simulink model "DriveTrainFinal"  (R2020b)
settings: Solver=VariableStepAuto  StartTime=0.0  StopTime=155  MaxStep=0.001  MinStep=0.0001  RelTol=1e-3
undefined symbols (not defined in the file): magnitude
libraries: simulink x3
settings Model: EnablePacing=on  Creator=markb  LastModifiedBy=orangejuzi
settings SolverCC: AlgebraicLoopSolver=LineSearch

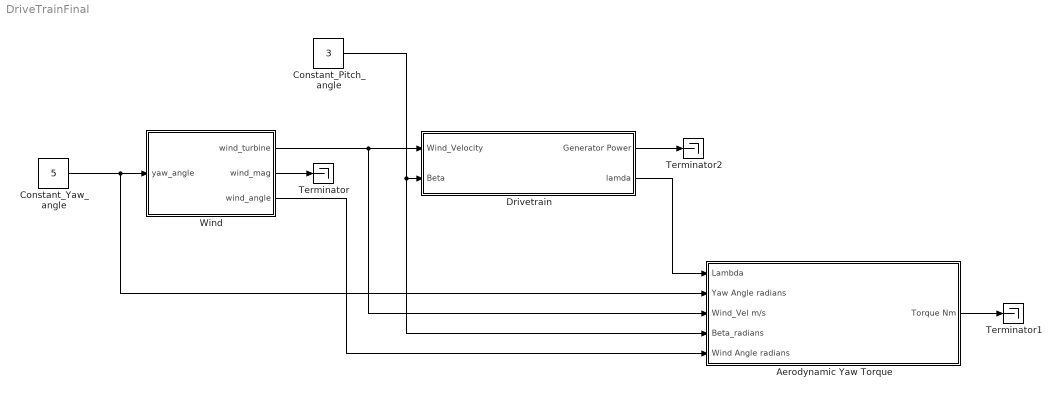
== system DriveTrainFinal ==
  Aerodynamic Yaw Torque : Subsystem
  Constant_Pitch_angle : Constant  Value=3
  Constant_Yaw_angle : Constant  Value=5
  Drivetrain : Subsystem
  Terminator : Terminator
  Terminator1 : Terminator
  Terminator2 : Terminator
  Wind : Subsystem
  wires:
  Wind/1(wind_turbine) -> Aerodynamic Yaw Torque/3(Wind_Vel m/s), Drivetrain/1(Wind_Velocity)
  Constant_Yaw_angle/1 -> Aerodynamic Yaw Torque/2(Yaw Angle radians), Wind/1(yaw_angle)
  Wind/2(wind_mag) -> Terminator/1
  Wind/3(wind_angle) -> Aerodynamic Yaw Torque/5(Wind Angle radians)
  Constant_Pitch_angle/1 -> Aerodynamic Yaw Torque/4(Beta_radians), Drivetrain/2(Beta)
  Drivetrain/1(Generator Power) -> Terminator2/1
  Drivetrain/2(lamda) -> Aerodynamic Yaw Torque/1(Lambda)
  Aerodynamic Yaw Torque/1(Torque Nm) -> Terminator1/1

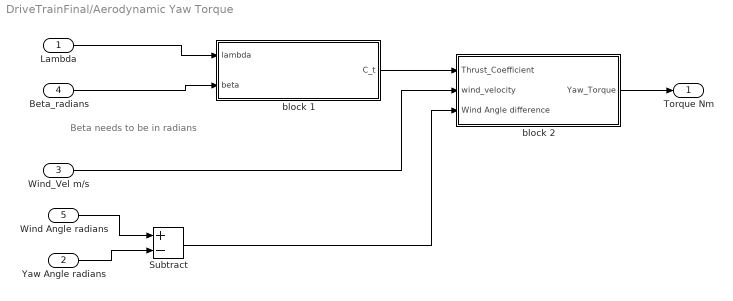
== system DriveTrainFinal/Aerodynamic Yaw Torque ==
  note: Beta needs to be in radians
  Lambda : Inport
  Yaw Angle radians : Inport  Port=2
  Wind_Vel m/s : Inport  Port=3
  Beta_radians : Inport  Port=4
  Wind Angle radians : Inport  Port=5
  Subtract : Sum  Inputs=+-
  block 1 : Subsystem
  block 2 : Subsystem
  Torque Nm : Outport
  wires:
  block 1/1(C_t) -> block 2/1(Thrust_Coefficient)
  Beta_radians/1 -> block 1/2(beta)
  Wind Angle radians/1 -> Subtract/1
  Yaw Angle radians/1 -> Subtract/2
  Subtract/1 -> block 2/3(Wind Angle difference)
  block 2/1(Yaw_Torque) -> Torque Nm/1
  Lambda/1 -> block 1/1(lambda)
  Wind_Vel m/s/1 -> block 2/2(wind_velocity)

== system DriveTrainFinal/Drivetrain ==
  Wind_Velocity : Inport
  Beta : Inport  Port=2
  Aerodynamic Block : Subsystem
  Electricl Block : Subsystem
  Mechanical Bock : Subsystem
  Generator Power : Outport
  lamda : Outport  Port=2
  wires:
  Mechanical Bock/2(omega_Gen) -> Electricl Block/1(HSS_Speed)
  Electricl Block/2(Generator Torque) -> Mechanical Bock/2(Gen_Torque)
  Mechanical Bock/1(omega_rotor) -> Aerodynamic Block/1(Rotor_Angular_Velocity)
  Wind_Velocity/1 -> Aerodynamic Block/2(Wind_Velocity)
  Beta/1 -> Aerodynamic Block/3(Beta)
  Aerodynamic Block/2(lamda) -> lamda/1
  Aerodynamic Block/1(Rotor_Torque) -> Mechanical Bock/1(Rotor_Torque)
  Electricl Block/1(Generator Power) -> Generator Power/1

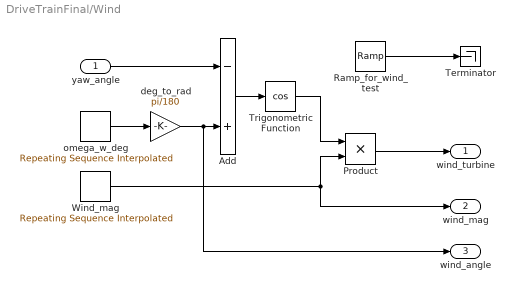
== system DriveTrainFinal/Wind ==
  yaw_angle : Inport
  Add : Sum  Inputs=-+
  Product : Product
  Ramp_for_wind_test : simulink/Sources/Ramp  slope=0.1  start=0  InitialOutput=10
  Terminator : Terminator
  Trigonometric Function : Trigonometry  Operator=cos
  Wind_mag : simulink/Sources/Repeating Sequence Interpolated  OutValues=[6 10 15 10 10 15 18 20 22 26 20 22 18 15 13 13 12 10 9 11 17 17 19 19 25 25 26 19 13 10 7 ].'  TimeValues=[0 5 15 20 25 30 35 40 45 50 55 60 65 70 75 80 85 90 95 100 105 110 115 120 125 130 135 140 145 150 155 ].'  LookUpMeth=Interpolation-Use End Values  tsamp=0.01  OutMin=[]  OutMax=[]  OutDataTypeStr=double  OutputDataTypeScalingMode=double  OutDataType=fixdt(0,8)  OutScaling=2^-10
  deg_to_rad : Gain  Gain=pi/180
  omega_w_deg : simulink/Sources/Repeating Sequence Interpolated  OutValues=[ 0 0 0 6 10 12 12 4 8 12 16 16 24 28 24 16 12 4 2 0 0 -2 -4 -4 -10 -14 -18 -20 -12 -8 -4 ].'  TimeValues=[0 5 15 20 25 30 35 40 45 50 55 60 65 70 75 80 85 90 95 100 105 110 115 120 125 130 135 140 145 150 155 ].'  LookUpMeth=Interpolation-Use End Values  tsamp=0.01  OutMin=[]  OutMax=[]  OutDataTypeStr=double  OutputDataTypeScalingMode=double  OutDataType=fixdt(0,8)  OutScaling=2^-10
  wind_turbine : Outport
  wind_mag : Outport  Port=2
  wind_angle : Outport  Port=3
  wires:
  Add/1 -> Trigonometric Function/1
  Trigonometric Function/1 -> Product/1
  deg_to_rad/1 -> wind_angle/1, Add/2
  yaw_angle/1 -> Add/1
  omega_w_deg/1 -> deg_to_rad/1
  Wind_mag/1 -> wind_mag/1, Product/2
  Product/1 -> wind_turbine/1
  Ramp_for_wind_test/1 -> Terminator/1

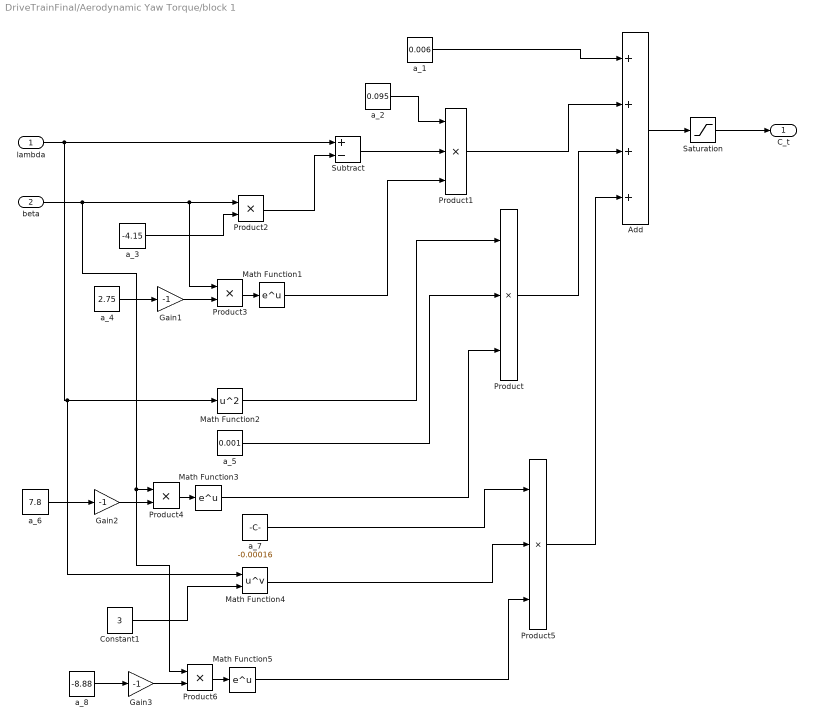
== system DriveTrainFinal/Aerodynamic Yaw Torque/block 1 ==
  lambda : Inport
  beta : Inport  Port=2
  Add : Sum  Inputs=++++
  Constant1 : Constant  Value=3
  Gain1 : Gain  Gain=-1
  Gain2 : Gain  Gain=-1
  Gain3 : Gain  Gain=-1
  Math Function1 : Math  SaturateOnIntegerOverflow=on
  Math Function2 : Math  Operator=square  SaturateOnIntegerOverflow=on
  Math Function3 : Math  SaturateOnIntegerOverflow=on
  Math Function4 : Math  Operator=pow  SaturateOnIntegerOverflow=on
  Math Function5 : Math  SaturateOnIntegerOverflow=on
  Product : Product  Inputs=3
  Product1 : Product  Inputs=3
  Product{2..4,6} (4 alike) : Product
  Product5 : Product  Inputs=3
  Saturation : Saturate  UpperLimit=inf  LowerLimit=0
  Subtract : Sum  Inputs=+-
  a_1 : Constant  Value=0.006
  a_2 : Constant  Value=0.095
  a_3 : Constant  Value=-4.15
  a_4 : Constant  Value=2.75
  a_5 : Constant  Value=0.001
  a_6 : Constant  Value=7.8
  a_7 : Constant  Value=-0.00016
  a_8 : Constant  Value=-8.88
  C_t : Outport
  wires:
  a_3/1 -> Product2/2
  beta/1 -> Product6/1, Product4/1, Product2/1, Product3/1
  a_1/1 -> Add/1
  Product1/1 -> Add/2
  Math Function5/1 -> Product5/3
  Gain3/1 -> Product6/2
  lambda/1 -> Math Function4/1, Math Function2/1, Subtract/1
  Math Function2/1 -> Product/1
  a_4/1 -> Gain1/1
  Product5/1 -> Add/4
  a_2/1 -> Product1/1
  Product3/1 -> Math Function1/1
  Product6/1 -> Math Function5/1
  Product4/1 -> Math Function3/1
  Math Function1/1 -> Product1/3
  Constant1/1 -> Math Function4/2
  Math Function4/1 -> Product5/2
  a_5/1 -> Product/2
  Add/1 -> Saturation/1
  Product2/1 -> Subtract/2
  Subtract/1 -> Product1/2
  Gain1/1 -> Product3/2
  a_7/1 -> Product5/1
  a_8/1 -> Gain3/1
  Gain2/1 -> Product4/2
  Math Function3/1 -> Product/3
  Product/1 -> Add/3
  a_6/1 -> Gain2/1
  Saturation/1 -> C_t/1

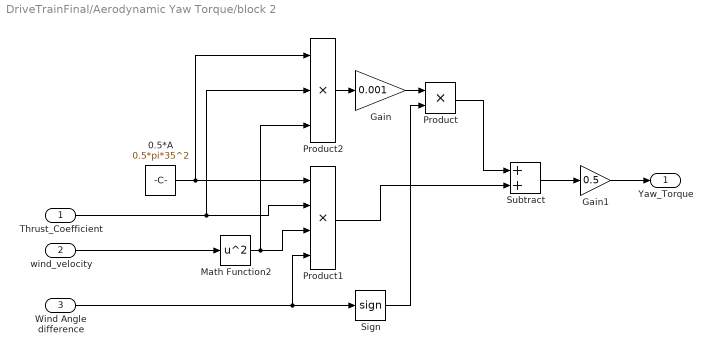
== system DriveTrainFinal/Aerodynamic Yaw Torque/block 2 ==
  Thrust_Coefficient : Inport
  wind_velocity : Inport  Port=2
  Wind Angle difference : Inport  Port=3
  0.5*A : Constant  Value=0.5*pi*35^2
  Gain : Gain  Gain=0.001
  Gain1 : Gain  Gain=0.5
  Math Function2 : Math  Operator=square  SaturateOnIntegerOverflow=on
  Product : Product
  Product1 : Product  Inputs=4
  Product2 : Product  Inputs=3
  Sign : Signum
  Subtract : Sum
  Yaw_Torque : Outport
  wires:
  0.5*A/1 -> Product2/1, Product1/1
  Thrust_Coefficient/1 -> Product2/2, Product1/2
  Math Function2/1 -> Product2/3, Product1/3
  wind_velocity/1 -> Math Function2/1
  Wind Angle difference/1 -> Product1/4, Sign/1
  Product2/1 -> Gain/1
  Product1/1 -> Subtract/2
  Subtract/1 -> Gain1/1
  Gain/1 -> Product/1
  Sign/1 -> Product/2
  Product/1 -> Subtract/1
  Gain1/1 -> Yaw_Torque/1

== system DriveTrainFinal/Drivetrain/Aerodynamic Block ==
  Rotor_Angular_Velocity : Inport
  Wind_Velocity : Inport  Port=2
  Beta : Inport  Port=3
  Power Coefficient : Subsystem
  Rotor Torque : Subsystem
  Tip speed Ratio : Subsystem
  Rotor_Torque : Outport
  lamda : Outport  Port=2
  wires:
  Beta/1 -> Power Coefficient/2(Beta)
  Tip speed Ratio/1(Tip_Speed_Ratio) -> lamda/1, Power Coefficient/1(Lamda)
  Power Coefficient/1(C_p) -> Rotor Torque/1(Power_Coefficient)
  Rotor_Angular_Velocity/1 -> Rotor Torque/3(Rotor_Angular_Velocity), Tip speed Ratio/1(Rotor_Angular_Velocity)
  Rotor Torque/1(Rotor_Torque) -> Rotor_Torque/1
  Wind_Velocity/1 -> Rotor Torque/2(Wind_Speed), Tip speed Ratio/2(Wind_Velocity)

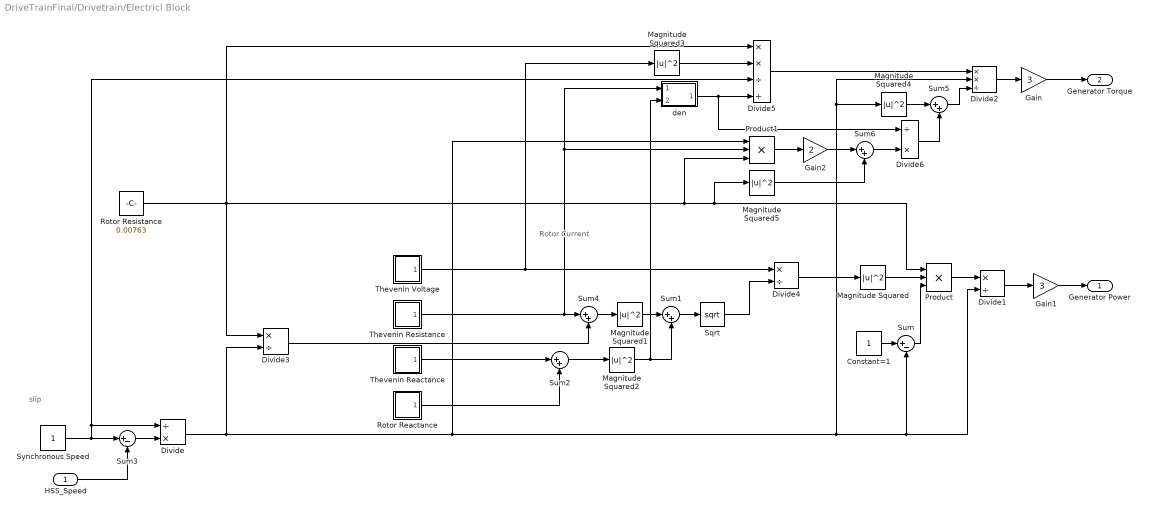
== system DriveTrainFinal/Drivetrain/Electricl Block ==
  note: slip
  note: Rotor Current
  HSS_Speed : Inport
  Constant=1 : Constant
  Divide : Product  Inputs=/*
  Divide1 : Product  Inputs=*/
  Divide2 : Product  Inputs=**/
  Divide3 : Product  Inputs=*/
  Divide4 : Product  Inputs=*/
  Divide5 : Product  Inputs=**//
  Divide6 : Product  Inputs=/*
  Gain : Gain  Gain=3
  Gain1 : Gain  Gain=3
  Gain2 : Gain  Gain=2
  Magnitude Squared{,1..5} (6 alike) : Math  Operator=magnitude^2  SaturateOnIntegerOverflow=on
  Product : Product  Inputs=3
  Product1 : Product  Inputs=3
  Rotor Reactance : Subsystem
  Rotor Resistance : Constant  Value=0.00763
  Sqrt : Sqrt  SaturateOnIntegerOverflow=on
  Sum : Sum  Inputs=|+-
  Sum{1..2,4..6} (5 alike) : Sum  Inputs=|++
  Sum3 : Sum  Inputs=|+-
  Synchronous Speed : Constant
  Thevenin Reactance : Subsystem
  Thevenin Resistance : Subsystem
  Thevenin Voltage : Subsystem
  den : Subsystem
  Generator Power : Outport
  Generator Torque : Outport  Port=2
  wires:
  Product/1 -> Divide1/1
  Divide1/1 -> Gain1/1
  Gain1/1 -> Generator Power/1
  Sum/1 -> Product/3
  Divide/1 -> Product1/1, Divide1/2, Sum/2, Divide2/2, Magnitude Squared4/1, Divide3/2
  Constant=1/1 -> Sum/1
  Rotor Resistance/1 -> Product1/3, Product/1, Magnitude Squared5/1, Divide3/1, Divide5/1
  Divide4/1 -> Magnitude Squared/1
  Magnitude Squared/1 -> Product/2
  Gain/1 -> Generator Torque/1
  Divide2/1 -> Gain/1
  Thevenin Voltage/1(Out1) -> Magnitude Squared3/1, Divide4/1
  Divide3/1 -> Sum4/2
  Magnitude Squared2/1 -> Sum1/2, den/2(In2)
  Magnitude Squared1/1 -> Sum1/1
  Sqrt/1 -> Divide4/2
  Sum2/1 -> Magnitude Squared2/1
  Thevenin Reactance/1(Out1) -> Sum2/1
  Sum1/1 -> Sqrt/1
  Magnitude Squared3/1 -> Divide5/2
  Synchronous Speed/1 -> Divide5/3, Divide/1, Sum3/1
  HSS_Speed/1 -> Sum3/2
  Sum3/1 -> Divide/2
  Divide5/1 -> Divide2/1
  den/1(Out1) -> Divide6/1, Divide5/4
  Sum4/1 -> Magnitude Squared1/1
  Sum5/1 -> Divide2/3
  Magnitude Squared4/1 -> Sum5/1
  Divide6/1 -> Sum5/2
  Sum6/1 -> Divide6/2
  Gain2/1 -> Sum6/1
  Product1/1 -> Gain2/1
  Magnitude Squared5/1 -> Sum6/2
  Rotor Reactance/1(Out1) -> Sum2/2
  Thevenin Resistance/1(Out1) -> Sum4/1, Product1/2, den/1(In1)

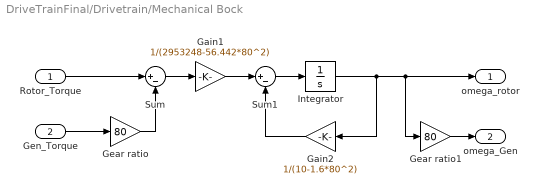
== system DriveTrainFinal/Drivetrain/Mechanical Bock ==
  Rotor_Torque : Inport
  Gen_Torque : Inport  Port=2
  Gain1 : Gain  Gain=1/(2953248-56.442*80^2)
  Gain2 : Gain  Gain=1/(10-1.6*80^2)
  Gear ratio : Gain  Gain=80
  Gear ratio1 : Gain  Gain=80
  Integrator : Integrator  InitialCondition=5
  Sum : Sum  Inputs=|+-
  Sum1 : Sum  Inputs=|+-
  omega_rotor : Outport
  omega_Gen : Outport  Port=2
  wires:
  Rotor_Torque/1 -> Sum/1
  Gen_Torque/1 -> Gear ratio/1
  Gear ratio/1 -> Sum/2
  Gain2/1 -> Sum1/2
  Gear ratio1/1 -> omega_Gen/1
  Sum1/1 -> Integrator/1
  Integrator/1 -> Gear ratio1/1, omega_rotor/1, Gain2/1
  Sum/1 -> Gain1/1
  Gain1/1 -> Sum1/1

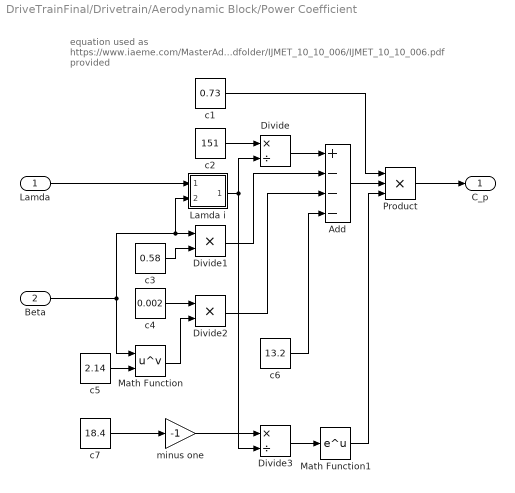
== system DriveTrainFinal/Drivetrain/Aerodynamic Block/Power Coefficient ==
  note: equation used as
      | https://www.iaeme.com/MasterAdmin/uploadfolder/IJMET_10_10_006/IJMET_10_10_006.pdf provided
  Lamda : Inport
  Beta : Inport  Port=2
  Add : Sum  Inputs=+---
  Divide : Product  Inputs=*/
  Divide1 : Product  Inputs=**
  Divide2 : Product  Inputs=**
  Divide3 : Product  Inputs=*/
  Lamda i : Subsystem
  Math Function : Math  Operator=pow  SaturateOnIntegerOverflow=on
  Math Function1 : Math  SaturateOnIntegerOverflow=on
  Product : Product  Inputs=3
  c1 : Constant  Value=0.73
  c2 : Constant  Value=151
  c3 : Constant  Value=0.58
  c4 : Constant  Value=0.002
  c5 : Constant  Value=2.14
  c6 : Constant  Value=13.2
  c7 : Constant  Value=18.4
  minus one : Gain  Gain=-1
  C_p : Outport
  wires:
  Lamda/1 -> Lamda i/1(In1)
  Beta/1 -> Math Function/1, Divide1/1, Lamda i/2(In2)
  c1/1 -> Product/1
  Product/1 -> C_p/1
  Add/1 -> Product/2
  c2/1 -> Divide/1
  Divide/1 -> Add/1
  Lamda i/1(Out1) -> Divide3/2, Divide/2
  c3/1 -> Divide1/2
  Divide1/1 -> Add/2
  c4/1 -> Divide2/1
  Math Function/1 -> Divide2/2
  c5/1 -> Math Function/2
  Divide2/1 -> Add/3
  c6/1 -> Add/4
  Divide3/1 -> Math Function1/1
  c7/1 -> minus one/1
  minus one/1 -> Divide3/1
  Math Function1/1 -> Product/3

== system DriveTrainFinal/Drivetrain/Aerodynamic Block/Rotor Torque ==
  note: Power of wind
  Power_Coefficient : Inport
  Wind_Speed : Inport  Port=2
  Rotor_Angular_Velocity : Inport  Port=3
  Divide : Product  Inputs=**/
  Gain : Gain  Gain=0.5*1.225*pi*35^2
  Product : Product
  Square : Math  Operator=square  SaturateOnIntegerOverflow=on
  Rotor_Torque : Outport
  wires:
  Rotor_Angular_Velocity/1 -> Divide/3  "omega_rotor"
  Power_Coefficient/1 -> Divide/1
  Divide/1 -> Rotor_Torque/1
  Wind_Speed/1 -> Square/1, Product/1  "V_wind"
  Gain/1 -> Divide/2
  Product/1 -> Gain/1
  Square/1 -> Product/2

== system DriveTrainFinal/Drivetrain/Aerodynamic Block/Tip speed Ratio ==
  Rotor_Angular_Velocity : Inport
  Wind_Velocity : Inport  Port=2
  Divide : Product  Inputs=*/
  Radius : Gain  Gain=35
  Tip_Speed_Ratio : Outport
  wires:
  Rotor_Angular_Velocity/1 -> Radius/1  "omega_r"
  Radius/1 -> Divide/1
  Wind_Velocity/1 -> Divide/2  "V_wind"
  Divide/1 -> Tip_Speed_Ratio/1

== system DriveTrainFinal/Drivetrain/Electricl Block/Rotor Reactance ==
  Gain3 : Gain  Gain=2*pi
  Rotor Inductance : Constant  Value=0.000195
  Out1 : Outport
  wires:
  Gain3/1 -> Out1/1
  Rotor Inductance/1 -> Gain3/1

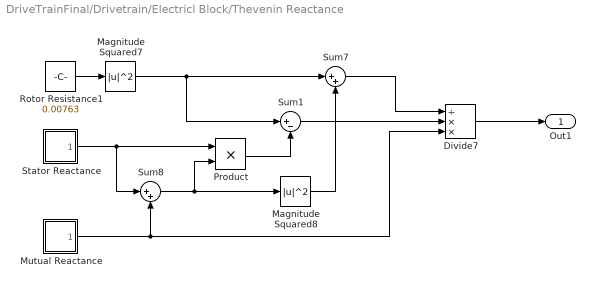
== system DriveTrainFinal/Drivetrain/Electricl Block/Thevenin Reactance ==
  Divide7 : Product  Inputs=/**
  Magnitude Squared7 : Math  Operator=magnitude^2  SaturateOnIntegerOverflow=on
  Magnitude Squared8 : Math  Operator=magnitude^2  SaturateOnIntegerOverflow=on
  Mutual Reactance : Subsystem
  Product : Product
  Rotor Resistance1 : Constant  Value=0.00763
  Stator Reactance : Subsystem
  Sum1 : Sum  Inputs=|+-
  Sum7 : Sum  Inputs=|++
  Sum8 : Sum  Inputs=|++
  Out1 : Outport
  wires:
  Sum7/1 -> Divide7/1
  Magnitude Squared7/1 -> Sum1/1, Sum7/1
  Divide7/1 -> Out1/1
  Stator Reactance/1(Out1) -> Product/1, Sum8/1
  Sum8/1 -> Product/2, Magnitude Squared8/1
  Rotor Resistance1/1 -> Magnitude Squared7/1
  Magnitude Squared8/1 -> Sum7/2
  Mutual Reactance/1(Out1) -> Divide7/3, Sum8/2
  Sum1/1 -> Divide7/2
  Product/1 -> Sum1/2

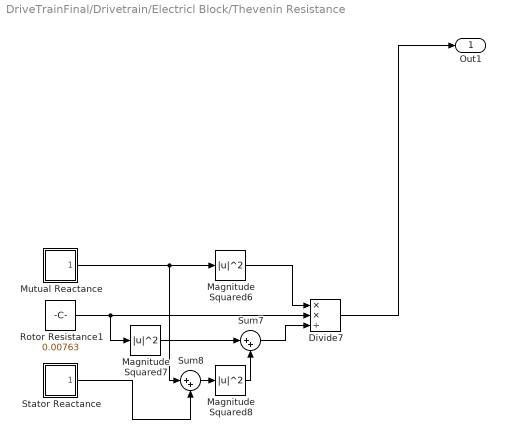
== system DriveTrainFinal/Drivetrain/Electricl Block/Thevenin Resistance ==
  Divide7 : Product  Inputs=**/
  Magnitude Squared6 : Math  Operator=magnitude^2  SaturateOnIntegerOverflow=on
  Magnitude Squared7 : Math  Operator=magnitude^2  SaturateOnIntegerOverflow=on
  Magnitude Squared8 : Math  Operator=magnitude^2  SaturateOnIntegerOverflow=on
  Mutual Reactance : Subsystem
  Rotor Resistance1 : Constant  Value=0.00763
  Stator Reactance : Subsystem
  Sum7 : Sum  Inputs=|++
  Sum8 : Sum  Inputs=|++
  Out1 : Outport
  wires:
  Sum7/1 -> Divide7/3
  Magnitude Squared7/1 -> Sum7/1
  Divide7/1 -> Out1/1
  Stator Reactance/1(Out1) -> Sum8/2
  Sum8/1 -> Magnitude Squared8/1
  Rotor Resistance1/1 -> Divide7/2, Magnitude Squared7/1
  Magnitude Squared6/1 -> Divide7/1
  Magnitude Squared8/1 -> Sum7/2
  Mutual Reactance/1(Out1) -> Sum8/1, Magnitude Squared6/1

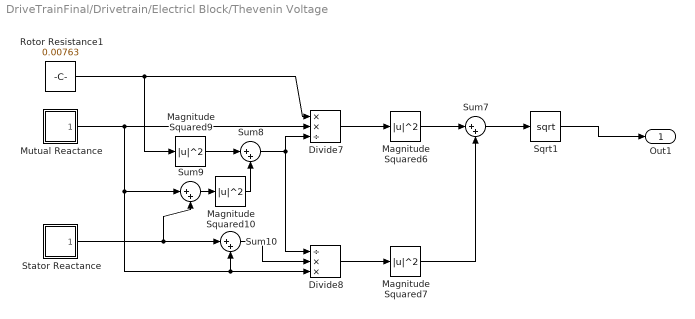
== system DriveTrainFinal/Drivetrain/Electricl Block/Thevenin Voltage ==
  Divide7 : Product  Inputs=**/
  Divide8 : Product  Inputs=/**
  Magnitude Squared{6..7,9..10} (4 alike) : Math  Operator=magnitude^2  SaturateOnIntegerOverflow=on
  Mutual Reactance : Subsystem
  Rotor Resistance1 : Constant  Value=0.00763
  Sqrt1 : Sqrt  SaturateOnIntegerOverflow=on
  Stator Reactance : Subsystem
  Sum{7..10} (4 alike) : Sum  Inputs=|++
  Out1 : Outport
  wires:
  Sum10/1 -> Divide8/2
  Sum7/1 -> Sqrt1/1
  Sqrt1/1 -> Out1/1
  Mutual Reactance/1(Out1) -> Divide7/2, Sum9/1, Sum10/2, Divide8/3
  Stator Reactance/1(Out1) -> Sum9/2, Sum10/1
  Sum9/1 -> Magnitude Squared10/1
  Magnitude Squared9/1 -> Sum8/1
  Divide8/1 -> Magnitude Squared7/1
  Sum8/1 -> Divide8/1, Divide7/3
  Magnitude Squared10/1 -> Sum8/2
  Magnitude Squared7/1 -> Sum7/2
  Magnitude Squared6/1 -> Sum7/1
  Rotor Resistance1/1 -> Divide7/1, Magnitude Squared9/1
  Divide7/1 -> Magnitude Squared6/1

== system DriveTrainFinal/Drivetrain/Electricl Block/den ==
  In1 : Inport
  In2 : Inport  Port=2
  Magnitude Squared4 : Math  Operator=magnitude^2  SaturateOnIntegerOverflow=on
  Sum4 : Sum  Inputs=|++
  Out1 : Outport
  wires:
  In2/1 -> Sum4/2
  In1/1 -> Magnitude Squared4/1
  Sum4/1 -> Out1/1
  Magnitude Squared4/1 -> Sum4/1

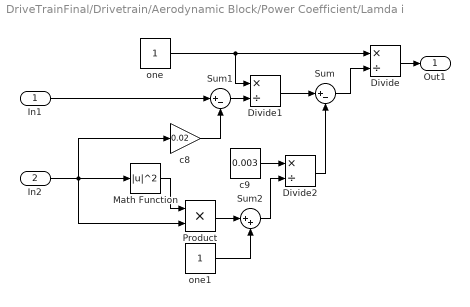
== system DriveTrainFinal/Drivetrain/Aerodynamic Block/Power Coefficient/Lamda i ==
  In1 : Inport
  In2 : Inport  Port=2
  Divide : Product  Inputs=*/
  Divide1 : Product  Inputs=*/
  Divide2 : Product  Inputs=*/
  Math Function : Math  Operator=magnitude^2  SaturateOnIntegerOverflow=on
  Product : Product
  Sum : Sum  Inputs=|+-
  Sum1 : Sum  Inputs=|+-
  Sum2 : Sum  Inputs=|++
  c8 : Gain  Gain=0.02
  c9 : Constant  Value=0.003
  one : Constant
  one1 : Constant
  Out1 : Outport
  wires:
  Divide/1 -> Out1/1
  In1/1 -> Sum1/1
  Product/1 -> Sum2/1
  Sum2/1 -> Divide2/2
  c8/1 -> Sum1/2
  Sum/1 -> Divide/2
  c9/1 -> Divide2/1
  Divide1/1 -> Sum/1
  Math Function/1 -> Product/1
  In2/1 -> Product/2, Math Function/1, c8/1
  one1/1 -> Sum2/2
  Divide2/1 -> Sum/2
  Sum1/1 -> Divide1/2
  one/1 -> Divide/1, Divide1/1

== system DriveTrainFinal/Drivetrain/Electricl Block/Thevenin Reactance/Mutual Reactance ==
  Gain3 : Gain  Gain=2*pi
  Mutual Inductance : Constant  Value=0.0007749
  Out1 : Outport
  wires:
  Gain3/1 -> Out1/1
  Mutual Inductance/1 -> Gain3/1

== system DriveTrainFinal/Drivetrain/Electricl Block/Thevenin Reactance/Stator Reactance ==
  Gain3 : Gain  Gain=2*pi
  Stator Inductance : Constant  Value=0.000195
  Out1 : Outport
  wires:
  Gain3/1 -> Out1/1
  Stator Inductance/1 -> Gain3/1

== system DriveTrainFinal/Drivetrain/Electricl Block/Thevenin Resistance/Mutual Reactance ==
  Gain3 : Gain  Gain=2*pi
  Mutual Inductance : Constant  Value=0.0007749
  Out1 : Outport
  wires:
  Gain3/1 -> Out1/1
  Mutual Inductance/1 -> Gain3/1

== system DriveTrainFinal/Drivetrain/Electricl Block/Thevenin Resistance/Stator Reactance ==
  Gain3 : Gain  Gain=2*pi
  Stator Inductance : Constant  Value=0.000195
  Out1 : Outport
  wires:
  Gain3/1 -> Out1/1
  Stator Inductance/1 -> Gain3/1

== system DriveTrainFinal/Drivetrain/Electricl Block/Thevenin Voltage/Mutual Reactance ==
  Gain3 : Gain  Gain=2*pi
  Mutual Inductance : Constant  Value=0.0007749
  Out1 : Outport
  wires:
  Gain3/1 -> Out1/1
  Mutual Inductance/1 -> Gain3/1

== system DriveTrainFinal/Drivetrain/Electricl Block/Thevenin Voltage/Stator Reactance ==
  Gain3 : Gain  Gain=2*pi
  Stator Inductance : Constant  Value=0.000195
  Out1 : Outport
  wires:
  Gain3/1 -> Out1/1
  Stator Inductance/1 -> Gain3/1
